simulink library "arc"  (R2023b)
settings: Solver=VariableStepAuto  StartTime=0.0  StopTime=10.0  RelTol=1e-3
values from neighbouring files (symbols this model uses):
  AF = 90    [BOTH_scenario_inputData.m]    (also in FC_scenario_inputData.m; PO_scenario_inputData.m = 0.7; inputData.m = 70; parametric_analysis_AF.m = AF_array(i))
  eta2 = 0.95    [BOTH_scenario_inputData.m]    (also in FC_scenario_inputData.m; PO_scenario_inputData.m; inputData.m; parametric_analysis_eta_tes.m = eta_tes_array(i))
  f51 = 0.33    [BOTH_scenario_inputData.m]    (also in FC_scenario_inputData.m; PO_scenario_inputData.m; inputData.m; worst_case_InputData.m)
  f53 = 0.33    [BOTH_scenario_inputData.m]    (also in FC_scenario_inputData.m; PO_scenario_inputData.m; inputData.m; worst_case_InputData.m)
  f54 = 1 - f51 - f53 - f56    (= 0.3399)    [BOTH_scenario_inputData.m]    (also in FC_scenario_inputData.m; PO_scenario_inputData.m; inputData.m; worst_case_InputData.m)
  f56 = 1e-4    (= 0.0001)    [BOTH_scenario_inputData.m]    (also in FC_scenario_inputData.m; PO_scenario_inputData.m; inputData.m; worst_case_InputData.m)
  f96 = 0.1    [BOTH_scenario_inputData.m]    (also in FC_scenario_inputData.m; PO_scenario_inputData.m; inputData.m; worst_case_InputData.m)
  f_dir = 0.7    [BOTH_scenario_inputData.m]    (also in FC_scenario_inputData.m; PO_scenario_inputData.m = 0.3; inputData.m = 0.3; parametric_analysis_f_dir.m = f_dir_array(i))
  f_permanent_trap = f_permanent_trap_array(i)    [parametric_analysis_trapping.m]
  fp3 = 1e-4    (= 0.0001)    [BOTH_scenario_inputData.m]    (also in FC_scenario_inputData.m; PO_scenario_inputData.m; inputData.m; parametric_analysis_f_p.m = f_p(i) / 2)
  fp4 = 1e-4    (= 0.0001)    [BOTH_scenario_inputData.m]    (also in FC_scenario_inputData.m; PO_scenario_inputData.m; inputData.m; parametric_analysis_f_p.m = f_p(i) / 2)
  I_s_0 = 1.85    [fuelCycleSimulator.m]    (also in parametric_analysis_AF.m = 0.8; parametric_analysis_epsi.m = 0.8; parametric_analysis_eta_tes.m = 0.8; parametric_analysis_f_dir.m = 0.8)
  lambda = 1.73e-9    (= 1.73e-09)    [BOTH_scenario_inputData.m]    (also in FC_scenario_inputData.m; PO_scenario_inputData.m; inputData.m; worst_case_InputData.m)
  M_structural = V_structural * rho_structural/1e3    (= 21350)    [inputData_trapping-lap-meschini.m]    (also in inputData_trapping.m = 27300)
  m_u = 1.6e-27    [inputData_trapping-lap-meschini.m]    (also in inputData_trapping.m)
  N_dot = 8.99e-7    (= 8.99e-07)    [BOTH_scenario_inputData.m]    (also in FC_scenario_inputData.m = 9.3e-07; PO_scenario_inputData.m = 9.3e-07; inputData.m = 9.3e-07; worst_case_InputData.m = 9.3e-07)
  n_structural = (rho_structural*1e3) / PM_structural * N_a    (= 7.36894684052e+25)    [inputData_trapping-lap-meschini.m]    (also in inputData_trapping.m = 8.4481294964e+28)
  n_trap = n_trap_array(j)    [parametric_analysis_trapping.m]
  n_trap_structural = n_trap_vcrti    (= 0.0001)    [inputData_trapping-lap-meschini.m]    (also in inputData_trapping.m = 0.000153880216982; parametric_analysis_trapping.m = n_trap_array(j))
  n_tungsten = (rho_tungsten*1e3) / PM_tungsten * N_a    (= 6.32342763874e+25)    [inputData_trapping-lap-meschini.m]    (also in inputData_trapping.m = 6.32342763874e+28)
  PM_structural = PM_vcrti    (= 49.85)    [inputData_trapping-lap-meschini.m]    (also in inputData_trapping.m = 55.6)
  PM_tritium = 3    [inputData_trapping-lap-meschini.m]    (also in inputData_trapping.m)
  T1 = 1/((1 + epsi)/tau1 + lambda)    [BOTH_scenario_inputData.m]    (also in FC_scenario_inputData.m; PO_scenario_inputData.m; inputData.m; parametric_analysis_epsi.m)
  T12 = 1/((1 + epsi)/tau12 + lambda)    [BOTH_scenario_inputData.m]    (also in FC_scenario_inputData.m; PO_scenario_inputData.m; inputData.m; parametric_analysis_epsi.m)
  T2 = 1/((1 + epsi)/tau2 + lambda)    [BOTH_scenario_inputData.m]    (also in FC_scenario_inputData.m; PO_scenario_inputData.m; inputData.m; parametric_analysis_epsi.m)
  T3 = 1/((1 + 0)/tau3 + lambda)    [BOTH_scenario_inputData.m]    (also in FC_scenario_inputData.m; PO_scenario_inputData.m; inputData.m; parametric_analysis_epsi.m)
  T4 = 1/((1 + 0)/tau4 + lambda)    [BOTH_scenario_inputData.m]    (also in FC_scenario_inputData.m; PO_scenario_inputData.m; inputData.m; parametric_analysis_epsi.m)
  T5 = 1/((1 + epsi)/tau5 + lambda)    [BOTH_scenario_inputData.m]    (also in FC_scenario_inputData.m; PO_scenario_inputData.m; inputData.m; parametric_analysis_epsi.m)
  T6 = 1/((1 + epsi)/tau6 + lambda)    [BOTH_scenario_inputData.m]    (also in FC_scenario_inputData.m; PO_scenario_inputData.m; inputData.m; parametric_analysis_epsi.m)
  T7 = 1/((1 + epsi)/tau7 + lambda)    [BOTH_scenario_inputData.m]    (also in FC_scenario_inputData.m; PO_scenario_inputData.m; inputData.m; parametric_analysis_epsi.m)
  T9 = 1/((1 + epsi)/tau9 + lambda)    [BOTH_scenario_inputData.m]    (also in FC_scenario_inputData.m; PO_scenario_inputData.m; inputData.m; parametric_analysis_TBE.m)
  tau1 = 1.25*3600    (= 4500)    [BOTH_scenario_inputData.m]    (also in FC_scenario_inputData.m; PO_scenario_inputData.m; inputData.m; parametric_analysis_t_blanket.m = tau1_array(i))
  tau12 = 100    [BOTH_scenario_inputData.m]    (also in FC_scenario_inputData.m; PO_scenario_inputData.m; inputData.m; worst_case_InputData.m)
  tau2 = 1*24*3600    (= 86400)    [BOTH_scenario_inputData.m]    (also in FC_scenario_inputData.m; PO_scenario_inputData.m; inputData.m; worst_case_InputData.m)
  tau3 = 1000    [BOTH_scenario_inputData.m]    (also in FC_scenario_inputData.m; PO_scenario_inputData.m; inputData.m; worst_case_InputData.m)
  tau4 = 1000    [BOTH_scenario_inputData.m]    (also in FC_scenario_inputData.m; PO_scenario_inputData.m; inputData.m; worst_case_InputData.m)
  tau5 = 1000    [BOTH_scenario_inputData.m]    (also in FC_scenario_inputData.m; PO_scenario_inputData.m; inputData.m; worst_case_InputData.m)
  tau6 = 3600    [BOTH_scenario_inputData.m]    (also in FC_scenario_inputData.m; PO_scenario_inputData.m; inputData.m; worst_case_InputData.m)
  tau7 = 600    [BOTH_scenario_inputData.m]    (also in FC_scenario_inputData.m; PO_scenario_inputData.m; inputData.m; worst_case_InputData.m)
  tau8 = 0.1*3600    (= 360)    [BOTH_scenario_inputData.m]    (also in FC_scenario_inputData.m; PO_scenario_inputData.m; inputData.m = 3600; parametric_analysis_TBE.m = t_p*0.1)
  tau9 = 0.9*3600    (= 3240)    [BOTH_scenario_inputData.m]    (also in FC_scenario_inputData.m; PO_scenario_inputData.m = 14040; inputData.m = 10800; parametric_analysis_TBE.m = t_p*0.9)
  tau_detrap_structural = 1 / nu_detrap_structural* relaxation_coefficient    [inputData_trapping-lap-meschini.m]    (also in inputData_trapping.m)
  tau_detrap_tungsten = 1 ./ nu_detrap* relaxation_coefficient    [inputData_trapping-lap-meschini.m]    (also in inputData_trapping.m)
  tau_trap_structural = 1/nu_trap_structural * relaxation_coefficient    [inputData_trapping-lap-meschini.m]    (also in inputData_trapping.m)
  TBE = 0.1    [BOTH_scenario_inputData.m]    (also in FC_scenario_inputData.m = 0.02; PO_scenario_inputData.m; inputData.m = 0.02; parametric_analysis_AF.m = TBE_array(j))
  TBR = 1.096    [fuelCycleSimulator.m]    (also in parametric_analysis_AF.m = 1; parametric_analysis_TBE.m = 1; parametric_analysis_epsi.m = 1; parametric_analysis_eta_tes.m = 1)
  V_structural = 3.5e6    (= 3500000)    [inputData_trapping-lap-meschini.m]    (also in inputData_trapping.m)
undefined symbols (not defined in the file or in its folder): f_permanent_trap_structural, n_solute, tau_detrap, tau_permanent, tau_permanent_structural, tau_trap
libraries: $bdroot x3, arc_2 x1
settings Model: Creator=smesc  LastModifiedBy=smesc
settings OptimizationCC: ReuseModelBlockBuffer=off
settings ModelReferenceCC: EnableRefExpFcnMdlSchedulingChecks=on

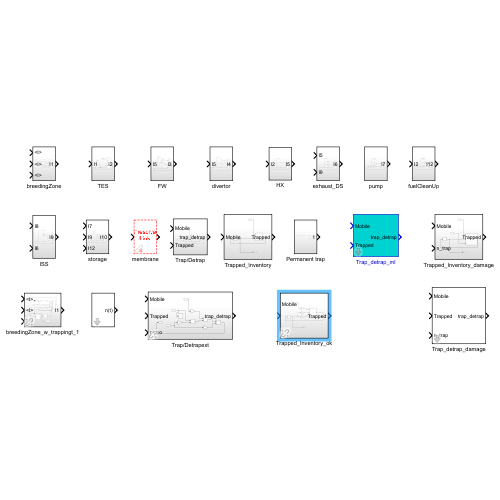
[thumbnail: Simulink's stored preview of the top-level diagram]
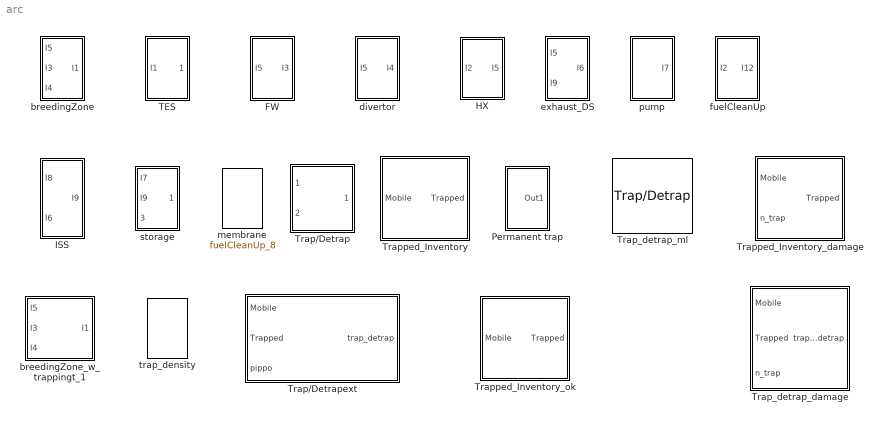
== system arc ==
  FW : Subsystem
      settings: LibrarySourceBlock=arc/FW_3
  HX : Subsystem
  ISS : Subsystem
      settings: LibrarySourceBlock=arc/ISS_9
  Permanent trap : Subsystem
  TES : Subsystem
      settings: LibrarySourceBlock=arc/TES_2
  Trap/Detrap : Subsystem
  Trap/Detrapext : Subsystem  AncestorBlock=arc/Trap//Detrap
  Trap_detrap_damage : Subsystem  mask{tau_trap=tau_trap_structural, tau_detrap=tau_detrap_tungsten(3), n_solute=n_solute, PM_host=PM_structural, PM_tritium=PM_tritium, M_host=M_structural}
      mask prompts: tau_trap "Tau trap"; tau_detrap "Tau detrap"; PM_host "PM host"; PM_tritium "PM T"
  Trap_detrap_ml : $bdroot/Trap//Detrap  mask{n_trap=0, tau_trap=0, tau_detrap=0, n_solute=0, PM_host=0, PM_tritium=0, M_host=0}
      mask prompts: n_trap "Trap density"; tau_trap "Tau trap"; tau_detrap "Tau detrap"; PM_host "PM host"; PM_tritium "PM T"
  Trapped_Inventory : Subsystem
  Trapped_Inventory_damage : Subsystem
  Trapped_Inventory_ok : Subsystem  AncestorBlock=arc/Trapped_Inventory
  breedingZone : Subsystem
      settings: LibrarySourceBlock=arc/breedingZone_1
  breedingZone_w_trappingt_1 : Subsystem  AncestorBlock=arc/breedingZone_1
      settings: LibrarySourceBlock=arc/breedingZone_1
  divertor : Subsystem
      settings: LibrarySourceBlock=arc/divertor_4
  exhaust_DS : Subsystem
  fuelCleanUp : Subsystem
      settings: LibrarySourceBlock=arc/fuelCleanUp_8
  membrane : $bdroot/fuelCleanUp_8  SystemSampleTime=-1  SSRTWFcnClass=[]  VariantActivationTime=update diagram  Latency=0  AutoFrameSizeCalculation=off
      settings: LibrarySourceBlock=arc/fuelCleanUp_8
  pump : Subsystem
      settings: LibrarySourceBlock=arc/pump_7
  storage : Subsystem
      settings: LibrarySourceBlock=arc/storage_10
  trap_density : arc_2/trap_density  n_max=1e-4  damage_rate=20/8760/3600  trap_creation_factor=1e28/n_tungsten  A_0=6.18e-3  E_annealing=0.38  T_material=950

== system arc/FW ==
  I5 : Inport
  Add : Sum  Inputs=++-
  Gain : Gain  Gain=f53/tau5
  Gain2 : Gain  Gain=1/T3
  Integrator : Integrator
  Pulse Generator : DiscretePulseGenerator  PulseType=Time based  Amplitude=fp3*N_dot/TBE  Period=1800  PulseWidth=AF
  I3 : Outport
  wires:
  I5/1 -> Gain/1
  Gain/1 -> Add/2
  Add/1 -> Integrator/1  "I_dot"
  Integrator/1 -> Gain2/1, I3/1  "I"
  Pulse Generator/1 -> Add/1
  Gain2/1 -> Add/3

== system arc/HX ==
  I2 : Inport
  Add : Sum  Inputs=+-
  Gain : Gain  Gain=(1-eta2)/tau2
  Gain3 : Gain  Gain=1/T5
  Integrator : Integrator
  I5 : Outport
  wires:
  I2/1 -> Gain/1
  Gain3/1 -> Add/2
  Gain/1 -> Add/1
  Add/1 -> Integrator/1  "I_dot"
  Integrator/1 -> I5/1, Gain3/1  "I"

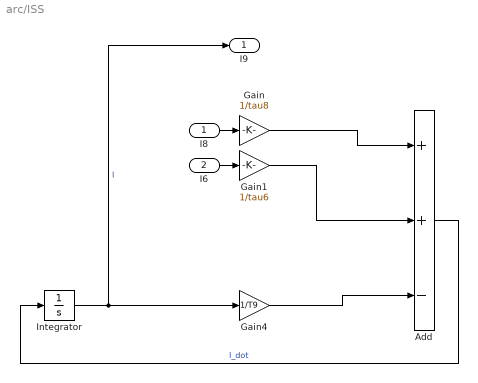
== system arc/ISS ==
  I8 : Inport
  I6 : Inport  Port=2
  Add : Sum  Inputs=++-
  Gain : Gain  Gain=1/tau8
  Gain1 : Gain  Gain=1/tau6
  Gain4 : Gain  Gain=1/T9
  Integrator : Integrator
  I9 : Outport
  wires:
  Gain4/1 -> Add/3
  Gain/1 -> Add/1
  Integrator/1 -> I9/1, Gain4/1  "I"
  Add/1 -> Integrator/1  "I_dot"
  I6/1 -> Gain1/1
  Gain1/1 -> Add/2
  I8/1 -> Gain/1

== system arc/Permanent trap ==
  Clock : Clock
  Exp : Math
  Gain1 : Gain  Gain=-1/tau_permanent
  Gain3 : Gain  Gain=f_permanent_trap*n_trap*n_tungsten*3*m_u*1/tau_permanent
  Scope : Scope
  Out1 : Outport
  wires:
  Exp/1 -> Gain3/1
  Gain3/1 -> Scope/1, Out1/1
  Clock/1 -> Gain1/1
  Gain1/1 -> Exp/1

== system arc/TES ==
  I1 : Inport
  Add : Sum  Inputs=+-
  Gain : Gain  Gain=1/T2
  Gain1 : Gain  Gain=1/tau1
  Integrator : Integrator
  Output : Outport
  wires:
  Add/1 -> Integrator/1  "I_dot"
  Integrator/1 -> Output/1, Gain/1  "I2"
  Gain1/1 -> Add/1
  I1/1 -> Gain1/1
  Gain/1 -> Add/2

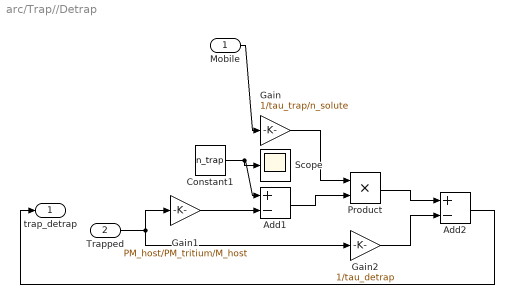
== system arc/Trap//Detrap ==
  Mobile : Inport
  Trapped : Inport  Port=2
  Add1 : Sum  Inputs=+-
  Add2 : Sum  Inputs=+-
  Constant1 : Constant  Value=n_trap
  Gain : Gain  Gain=1/tau_trap/n_solute
  Gain1 : Gain  Gain=PM_host/PM_tritium/M_host
  Gain2 : Gain  Gain=1/tau_detrap
  Product : Product
  Scope : Scope
  trap_detrap : Outport
  wires:
  Product/1 -> Add2/1
  Add2/1 -> trap_detrap/1
  Mobile/1 -> Gain/1
  Gain/1 -> Product/1
  Constant1/1 -> Scope/1, Add1/1
  Gain2/1 -> Add2/2
  Add1/1 -> Product/2
  Gain1/1 -> Add1/2
  Trapped/1 -> Gain2/1, Gain1/1

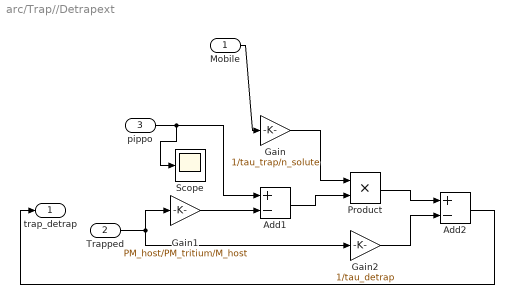
== system arc/Trap//Detrapext ==
  Mobile : Inport
  Trapped : Inport  Port=2
  pippo : Inport  Port=3
  Add1 : Sum  Inputs=+-
  Add2 : Sum  Inputs=+-
  Gain : Gain  Gain=1/tau_trap/n_solute
  Gain1 : Gain  Gain=PM_host/PM_tritium/M_host
  Gain2 : Gain  Gain=1/tau_detrap
  Product : Product
  Scope : Scope
  trap_detrap : Outport
  wires:
  Product/1 -> Add2/1
  Add2/1 -> trap_detrap/1
  Mobile/1 -> Gain/1
  Gain/1 -> Product/1
  pippo/1 -> Scope/1, Add1/1
  Gain2/1 -> Add2/2
  Add1/1 -> Product/2
  Gain1/1 -> Add1/2
  Trapped/1 -> Gain2/1, Gain1/1

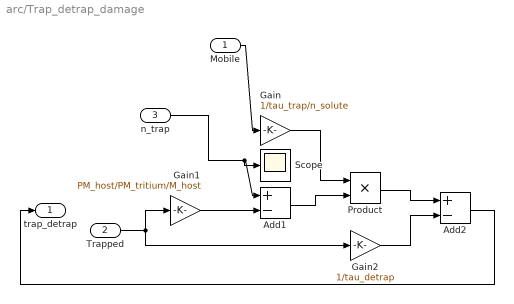
== system arc/Trap_detrap_damage ==
  Mobile : Inport
  Trapped : Inport  Port=2
  n_trap : Inport  Port=3
  Add1 : Sum  Inputs=+-
  Add2 : Sum  Inputs=+-
  Gain : Gain  Gain=1/tau_trap/n_solute
  Gain1 : Gain  Gain=PM_host/PM_tritium/M_host
  Gain2 : Gain  Gain=1/tau_detrap
  Product : Product
  Scope : Scope
  trap_detrap : Outport
  wires:
  Product/1 -> Add2/1
  Add2/1 -> trap_detrap/1
  Mobile/1 -> Gain/1
  Gain/1 -> Product/1
  n_trap/1 -> Scope/1, Add1/1
  Gain2/1 -> Add2/2
  Add1/1 -> Product/2
  Gain1/1 -> Add1/2
  Trapped/1 -> Gain2/1, Gain1/1

== system arc/Trapped_Inventory ==
  Mobile : Inport
  Integrator1 : Integrator
  Trap/Detrap : Subsystem
  Trapped : Outport
  wires:
  Integrator1/1 -> Trapped/1, Trap/Detrap/2(In2)
  Mobile/1 -> Trap/Detrap/1(In1)
  Trap/Detrap/1(Out1) -> Integrator1/1

== system arc/Trapped_Inventory_damage ==
  Mobile : Inport
  n_trap : Inport  Port=2
  Integrator1 : Integrator
  Trap_detrap_damage : $bdroot/Trap_detrap_damage  tau_trap=tau_trap_structural  tau_detrap=tau_detrap_tungsten(3)  n_solute=n_solute  PM_host=PM_structural  PM_tritium=PM_tritium  M_host=M_structural
  Trapped : Outport
  wires:
  Integrator1/1 -> Trap_detrap_damage/2, Trapped/1
  Mobile/1 -> Trap_detrap_damage/1
  Trap_detrap_damage/1 -> Integrator1/1
  n_trap/1 -> Trap_detrap_damage/3

== system arc/Trapped_Inventory_ok ==
  Mobile : Inport
  Add : Sum  Inputs=+--
  Gain : Gain  Gain=1/tau_trap
  Gain1 : Gain  Gain=1/tau_detrap
  Gain2 : Gain  Gain=lambda
  Integrator1 : Integrator
  Trapped : Outport
  wires:
  Integrator1/1 -> Trapped/1, Gain2/1, Gain1/1
  Mobile/1 -> Gain/1
  Add/1 -> Integrator1/1
  Gain/1 -> Add/1
  Gain2/1 -> Add/2
  Gain1/1 -> Add/3

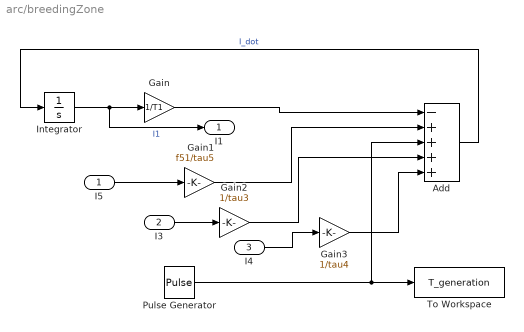
== system arc/breedingZone ==
  I5 : Inport
  I3 : Inport  Port=2
  I4 : Inport  Port=3
  Add : Sum  Inputs=-++++
  Gain : Gain  Gain=1/T1
  Gain1 : Gain  Gain=f51/tau5
  Gain2 : Gain  Gain=1/tau3
  Gain3 : Gain  Gain=1/tau4
  Integrator : Integrator
  Pulse Generator : DiscretePulseGenerator  PulseType=Time based  Amplitude=N_dot * TBR  Period=1800  PulseWidth=AF
  To Workspace : ToWorkspace  VariableName=T_generation  SaveFormat=Timeseries  SampleTime=-1
  I1 : Outport
  wires:
  Gain3/1 -> Add/5
  I4/1 -> Gain3/1
  Gain2/1 -> Add/4
  I3/1 -> Gain2/1
  Pulse Generator/1 -> To Workspace/1, Add/3
  I5/1 -> Gain1/1
  Gain/1 -> Add/1
  Integrator/1 -> I1/1, Gain/1  "I1"
  Gain1/1 -> Add/2
  Add/1 -> Integrator/1  "I_dot"

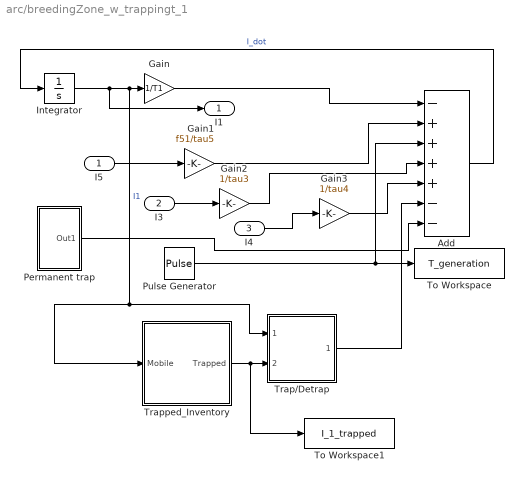
== system arc/breedingZone_w_trappingt_1 ==
  I5 : Inport
  I3 : Inport  Port=2
  I4 : Inport  Port=3
  Add : Sum  Inputs=-++++--
  Gain : Gain  Gain=1/T1
  Gain1 : Gain  Gain=f51/tau5
  Gain2 : Gain  Gain=1/tau3
  Gain3 : Gain  Gain=1/tau4
  Integrator : Integrator
  Permanent trap : Subsystem
  Pulse Generator : DiscretePulseGenerator  PulseType=Time based  Amplitude=N_dot * TBR  Period=1800  PulseWidth=AF
  To Workspace : ToWorkspace  VariableName=T_generation  SaveFormat=Timeseries  SampleTime=-1
  To Workspace1 : ToWorkspace  VariableName=I_1_trapped  SampleTime=-1
  Trap/Detrap : Subsystem  AncestorBlock=arc/Trap//Detrap
  Trapped_Inventory : Subsystem  AncestorBlock=arc/Trapped_Inventory
  I1 : Outport
  wires:
  Add/1 -> Integrator/1  "I_dot"
  Gain1/1 -> Add/2
  Integrator/1 -> Trapped_Inventory/1(Mobile), Trap/Detrap/1(Mobile), Gain/1, I1/1  "I1"
  Gain/1 -> Add/1
  I5/1 -> Gain1/1
  Pulse Generator/1 -> Add/3, To Workspace/1
  I3/1 -> Gain2/1
  Gain2/1 -> Add/4
  I4/1 -> Gain3/1
  Gain3/1 -> Add/5
  Trapped_Inventory/1(Trapped) -> To Workspace1/1, Trap/Detrap/2(Trapped)
  Trap/Detrap/1(trap_detrap) -> Add/6
  Permanent trap/1(Out1) -> Add/7

== system arc/divertor ==
  I5 : Inport
  Add : Sum  Inputs=++-
  Gain : Gain  Gain=f54/tau5
  Gain2 : Gain  Gain=1/T4
  Integrator : Integrator
  Pulse Generator : DiscretePulseGenerator  PulseType=Time based  Amplitude=fp4*N_dot/TBE  Period=1800  PulseWidth=AF
  I4 : Outport
  wires:
  I5/1 -> Gain/1
  Gain2/1 -> Add/3
  Add/1 -> Integrator/1  "I_dot"
  Integrator/1 -> I4/1, Gain2/1  "I"
  Gain/1 -> Add/2
  Pulse Generator/1 -> Add/1

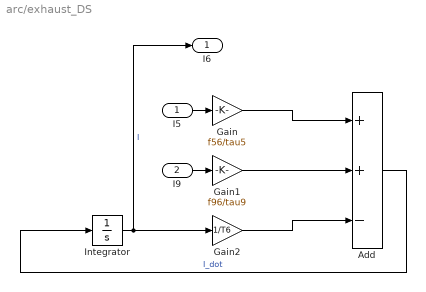
== system arc/exhaust_DS ==
  I5 : Inport
  I9 : Inport  Port=2
  Add : Sum  Inputs=++-
  Gain : Gain  Gain=f56/tau5
  Gain1 : Gain  Gain=f96/tau9
  Gain2 : Gain  Gain=1/T6
  Integrator : Integrator
  I6 : Outport
  wires:
  Gain/1 -> Add/1
  I5/1 -> Gain/1
  Gain1/1 -> Add/2
  Add/1 -> Integrator/1  "I_dot"
  Gain2/1 -> Add/3
  Integrator/1 -> I6/1, Gain2/1  "I"
  I9/1 -> Gain1/1

== system arc/fuelCleanUp ==
  I2 : Inport
  Add : Sum  Inputs=+-
  Gain : Gain  Gain=eta2/tau2
  Gain1 : Gain  Gain=1/T12
  Integrator : Integrator
  I12 : Outport
  wires:
  Gain/1 -> Add/1
  Integrator/1 -> I12/1, Gain1/1  "I"
  Add/1 -> Integrator/1  "I_dot"
  Gain1/1 -> Add/2
  I2/1 -> Gain/1

== system arc/pump ==
  Add : Sum  Inputs=+-
  Gain : Gain  Gain=1/T7
  Integrator : Integrator
  Pulse Generator : DiscretePulseGenerator  PulseType=Time based  Amplitude=(1-TBE-fp3-fp4)*N_dot/TBE  Period=1800  PulseWidth=AF
  I7 : Outport
  wires:
  Add/1 -> Integrator/1  "I_dot"
  Pulse Generator/1 -> Add/1
  Integrator/1 -> I7/1, Gain/1  "I7"
  Gain/1 -> Add/2

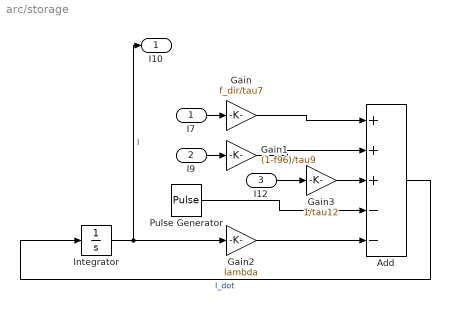
== system arc/storage ==
  I7 : Inport
  I9 : Inport  Port=2
  I12 : Inport  Port=3
  Add : Sum  Inputs=+++--
  Gain : Gain  Gain=f_dir/tau7
  Gain1 : Gain  Gain=(1-f96)/tau9
  Gain2 : Gain  Gain=lambda
  Gain3 : Gain  Gain=1/tau12
  Integrator : Integrator  InitialCondition=I_s_0
  Pulse Generator : DiscretePulseGenerator  PulseType=Time based  Amplitude=N_dot/TBE  Period=1800  PulseWidth=AF
  I10 : Outport
  wires:
  Gain3/1 -> Add/3
  I12/1 -> Gain3/1
  Pulse Generator/1 -> Add/4
  Gain/1 -> Add/1
  Gain1/1 -> Add/2
  I7/1 -> Gain/1
  Gain2/1 -> Add/5
  Add/1 -> Integrator/1  "I_dot"
  I9/1 -> Gain1/1
  Integrator/1 -> I10/1, Gain2/1  "I"

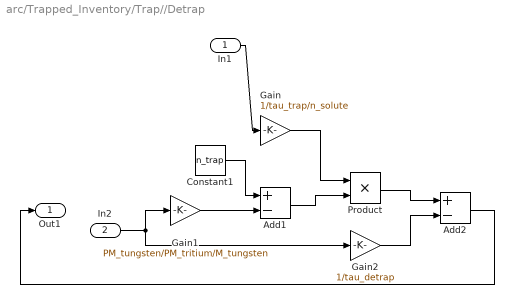
== system arc/Trapped_Inventory/Trap//Detrap ==
  In1 : Inport
  In2 : Inport  Port=2
  Add1 : Sum  Inputs=+-
  Add2 : Sum  Inputs=+-
  Constant1 : Constant  Value=n_trap
  Gain : Gain  Gain=1/tau_trap/n_solute
  Gain1 : Gain  Gain=PM_tungsten/PM_tritium/M_tungsten
  Gain2 : Gain  Gain=1/tau_detrap
  Product : Product
  Out1 : Outport
  wires:
  Product/1 -> Add2/1
  Add2/1 -> Out1/1
  In1/1 -> Gain/1
  Gain/1 -> Product/1
  Constant1/1 -> Add1/1
  Gain2/1 -> Add2/2
  Add1/1 -> Product/2
  Gain1/1 -> Add1/2
  In2/1 -> Gain2/1, Gain1/1

== system arc/breedingZone_w_trappingt_1/Permanent trap ==
  Add : Sum  Inputs=+-
  Clock : Clock
  Constant : Constant
  Exp : Math
  Gain1 : Gain  Gain=-1/tau_permanent_structural
  Gain3 : Gain  Gain=f_permanent_trap_structural*n_trap_structural*n_structural*3*m_u*1*(V_structural/2)
  Scope : Scope
  Out1 : Outport
  wires:
  Gain3/1 -> Scope/1, Out1/1
  Clock/1 -> Gain1/1
  Gain1/1 -> Exp/1
  Add/1 -> Gain3/1
  Constant/1 -> Add/1
  Exp/1 -> Add/2

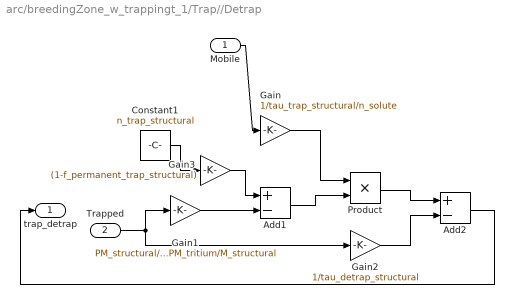
== system arc/breedingZone_w_trappingt_1/Trap//Detrap ==
  Mobile : Inport
  Trapped : Inport  Port=2
  Add1 : Sum  Inputs=+-
  Add2 : Sum  Inputs=+-
  Constant1 : Constant  Value=n_trap_structural
  Gain : Gain  Gain=1/tau_trap_structural/n_solute
  Gain1 : Gain  Gain=PM_structural/PM_tritium/M_structural
  Gain2 : Gain  Gain=1/tau_detrap_structural
  Gain3 : Gain  Gain=(1-f_permanent_trap_structural)
  Product : Product
  trap_detrap : Outport
  wires:
  Trapped/1 -> Gain1/1, Gain2/1
  Gain1/1 -> Add1/2
  Add1/1 -> Product/2
  Gain2/1 -> Add2/2
  Gain/1 -> Product/1
  Mobile/1 -> Gain/1
  Add2/1 -> trap_detrap/1
  Product/1 -> Add2/1
  Constant1/1 -> Gain3/1
  Gain3/1 -> Add1/1

== system arc/breedingZone_w_trappingt_1/Trapped_Inventory ==
  Mobile : Inport
  Integrator1 : Integrator
  Trap/Detrap : Subsystem
  Trapped : Outport
  wires:
  Trap/Detrap/1(Out1) -> Integrator1/1
  Mobile/1 -> Trap/Detrap/1(In1)
  Integrator1/1 -> Trap/Detrap/2(In2), Trapped/1

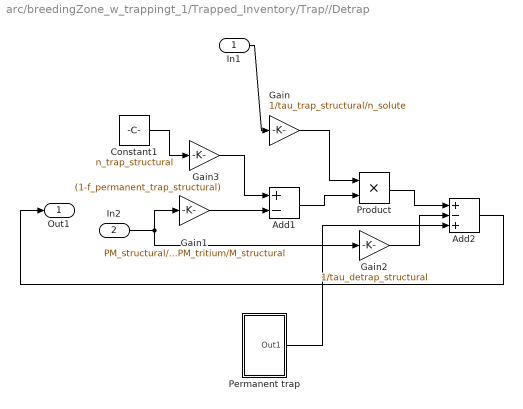
== system arc/breedingZone_w_trappingt_1/Trapped_Inventory/Trap//Detrap ==
  In1 : Inport
  In2 : Inport  Port=2
  Add1 : Sum  Inputs=+-
  Add2 : Sum  Inputs=+-+
  Constant1 : Constant  Value=n_trap_structural
  Gain : Gain  Gain=1/tau_trap_structural/n_solute
  Gain1 : Gain  Gain=PM_structural/PM_tritium/M_structural
  Gain2 : Gain  Gain=1/tau_detrap_structural
  Gain3 : Gain  Gain=(1-f_permanent_trap_structural)
  Permanent trap : Subsystem
  Product : Product
  Out1 : Outport
  wires:
  In2/1 -> Gain1/1, Gain2/1
  Gain1/1 -> Add1/2
  Add1/1 -> Product/2
  Gain2/1 -> Add2/2
  Gain/1 -> Product/1
  In1/1 -> Gain/1
  Add2/1 -> Out1/1
  Product/1 -> Add2/1
  Permanent trap/1(Out1) -> Add2/3
  Constant1/1 -> Gain3/1
  Gain3/1 -> Add1/1

== system arc/breedingZone_w_trappingt_1/Trapped_Inventory/Trap//Detrap/Permanent trap ==
  Add : Sum  Inputs=+-
  Clock : Clock
  Constant : Constant
  Exp : Math
  Gain1 : Gain  Gain=-1/tau_permanent_structural
  Gain3 : Gain  Gain=f_permanent_trap_structural*n_trap_structural*n_structural*3*m_u*1*(V_structural/2)
  Scope : Scope
  Out1 : Outport
  wires:
  Gain3/1 -> Scope/1, Out1/1
  Clock/1 -> Gain1/1
  Gain1/1 -> Exp/1
  Add/1 -> Gain3/1
  Constant/1 -> Add/1
  Exp/1 -> Add/2
